simulink model "AdaptiveOb"  (R2019b)
settings: Solver=VariableStepAuto  StartTime=0.0  StopTime=10.0  RelTol=1e-3
undefined symbols (not defined in the file): DiscIntNeverNeededParam, INJ_FRQ, J, KLdd, KLgd, KLgg, KR, Ldq, LGammaDelta, RsRated, theta_tilde, TsimCurLoop, TsimMotor, Umdh_Cmd, Umgh_Cmd, weRated
settings Model: Creator=Downstream  LastModifiedBy=Downstream

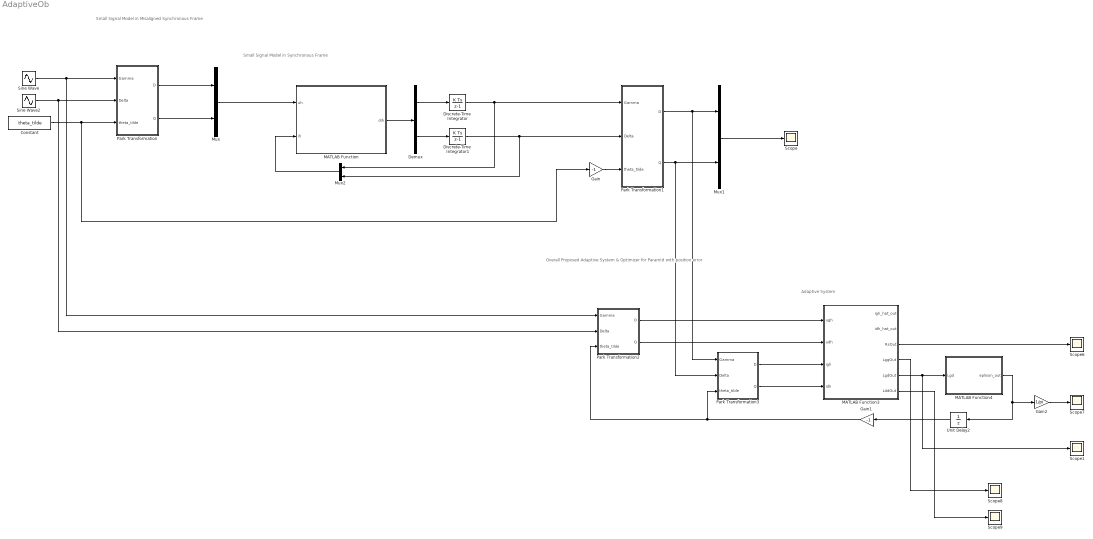
== system AdaptiveOb ==
  note: Overall Proposed Adaptive System & Optimizer for ParamId with position error
  note: Adaptive System
  note: Small Signal Model in Misaligned Synchronous Frame
  note: Small Signal Model in Synchronous Frame
  Constant : Constant  Value=theta_tilde  SampleTime=TsimMotor
  Demux : Demux  Outputs=2
  Discrete-Time Integrator : DiscreteIntegrator  Priority=1  SampleTime=-1  ICPrevOutput=DiscIntNeverNeededParam  ICPrevScaledInput=DiscIntNeverNeededParam
  Discrete-Time Integrator1 : DiscreteIntegrator  Priority=1  SampleTime=-1  ICPrevOutput=DiscIntNeverNeededParam  ICPrevScaledInput=DiscIntNeverNeededParam
  Gain : Gain  Gain=-1
  Gain1 : Gain  Gain=-1
  Gain2 : Gain  Gain=1/pi
  MATLAB Function : MATLAB Function  TreatAsAtomicUnit=on
  MATLAB Function3 : MATLAB Function  Priority=9  TreatAsAtomicUnit=on  SystemSampleTime=TsimCurLoop
  MATLAB Function4 : MATLAB Function  TreatAsAtomicUnit=on
  Mux : Mux  Inputs=2
  Mux1 : Mux  Inputs=2
  Mux2 : Mux  Inputs=2
  Park Transformation : Subsystem
  Park Transformation1 : Subsystem
  Park Transformation2 : Subsystem
  Park Transformation3 : Subsystem
  Scope{,1,6..9} (6 alike) : Scope
  Sine Wave : Sin  Priority=4  Amplitude=Umgh_Cmd  Frequency=INJ_FRQ * 2 * pi  SampleTime=TsimCurLoop
  Sine Wave2 : Sin  Priority=5  Amplitude=Umdh_Cmd  Frequency=INJ_FRQ * 2 * pi  Phase=pi/2  SampleTime=TsimCurLoop
  Unit Delay2 : UnitDelay  SampleTime=-1  HasFrameUpgradeWarning=on
  wires:
  Constant/1 -> Park Transformation/3(theta_tilde), Gain/1
  Mux/1 -> MATLAB Function/1(uh)
  MATLAB Function/1(dih) -> Demux/1
  Demux/1 -> Discrete-Time Integrator/1
  Demux/2 -> Discrete-Time Integrator1/1
  Gain/1 -> Park Transformation1/3(theta_tilde)
  Mux1/1 -> Scope/1
  Park Transformation/1(D) -> Mux/1
  Park Transformation/2(Q) -> Mux/2
  Discrete-Time Integrator1/1 -> Park Transformation1/2(Delta), Mux2/2
  Discrete-Time Integrator/1 -> Mux2/1, Park Transformation1/1(Gamma)
  Mux2/1 -> MATLAB Function/2(ih)
  Park Transformation3/1(D) -> MATLAB Function3/3(igh)
  Park Transformation3/2(Q) -> MATLAB Function3/4(idh)
  MATLAB Function3/5(LgdOut) -> Scope1/1, MATLAB Function4/1(Lgd)
  MATLAB Function4/1(eplison_out) -> Gain2/1, Unit Delay2/1
  Gain1/1 -> Park Transformation3/3(theta_tilde), Park Transformation2/3(theta_tilde)
  MATLAB Function3/3(RsOut) -> Scope6/1
  Unit Delay2/1 -> Gain1/1
  Gain2/1 -> Scope7/1
  Sine Wave/1 -> Park Transformation2/1(Gamma), Park Transformation/1(Gamma)
  Sine Wave2/1 -> Park Transformation2/2(Delta), Park Transformation/2(Delta)
  MATLAB Function3/4(LggOut) -> Scope8/1
  MATLAB Function3/6(LddOut) -> Scope9/1
  Park Transformation1/1(D) -> Park Transformation3/1(Gamma), Mux1/1
  Park Transformation1/2(Q) -> Mux1/2, Park Transformation3/2(Delta)
  Park Transformation2/1(D) -> MATLAB Function3/1(ugh)
  Park Transformation2/2(Q) -> MATLAB Function3/2(udh)

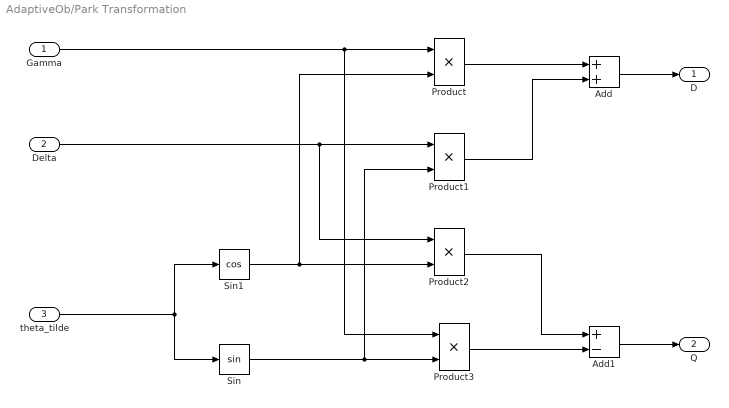
== system AdaptiveOb/Park Transformation ==
  Gamma : Inport
  Delta : Inport  Port=2
  theta_tilde : Inport  Port=3
  Add : Sum
  Add1 : Sum  Inputs=+-
  Product{,1..3} (4 alike) : Product
  Sin : Trigonometry  OutputSignalType=real
  Sin1 : Trigonometry  Operator=cos  OutputSignalType=real
  D : Outport
  Q : Outport  Port=2
  wires:
  Product/1 -> Add/1
  Sin/1 -> Product3/2, Product1/2
  Product1/1 -> Add/2
  Add1/1 -> Q/1
  Sin1/1 -> Product2/2, Product/2
  Product2/1 -> Add1/1
  Gamma/1 -> Product3/1, Product/1
  Delta/1 -> Product2/1, Product1/1
  Product3/1 -> Add1/2
  Add/1 -> D/1
  theta_tilde/1 -> Sin/1, Sin1/1

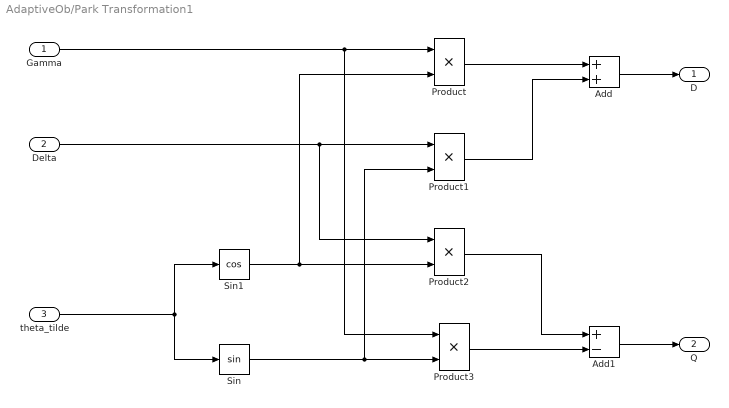
== system AdaptiveOb/Park Transformation1 ==
  Gamma : Inport
  Delta : Inport  Port=2
  theta_tilde : Inport  Port=3
  Add : Sum
  Add1 : Sum  Inputs=+-
  Product{,1..3} (4 alike) : Product
  Sin : Trigonometry  OutputSignalType=real
  Sin1 : Trigonometry  Operator=cos  OutputSignalType=real
  D : Outport
  Q : Outport  Port=2
  wires:
  Product/1 -> Add/1
  Sin/1 -> Product3/2, Product1/2
  Product1/1 -> Add/2
  Add1/1 -> Q/1
  Sin1/1 -> Product2/2, Product/2
  Product2/1 -> Add1/1
  Gamma/1 -> Product3/1, Product/1
  Delta/1 -> Product2/1, Product1/1
  Product3/1 -> Add1/2
  Add/1 -> D/1
  theta_tilde/1 -> Sin/1, Sin1/1

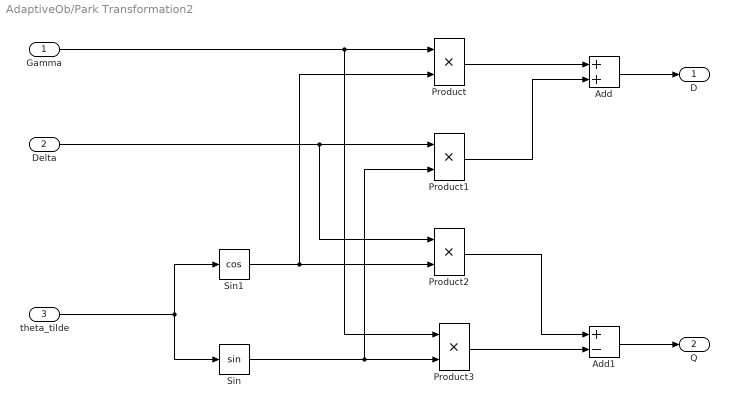
== system AdaptiveOb/Park Transformation2 ==
  Gamma : Inport
  Delta : Inport  Port=2
  theta_tilde : Inport  Port=3
  Add : Sum
  Add1 : Sum  Inputs=+-
  Product{,1..3} (4 alike) : Product
  Sin : Trigonometry  OutputSignalType=real
  Sin1 : Trigonometry  Operator=cos  OutputSignalType=real
  D : Outport
  Q : Outport  Port=2
  wires:
  Product/1 -> Add/1
  Sin/1 -> Product3/2, Product1/2
  Product1/1 -> Add/2
  Add1/1 -> Q/1
  Sin1/1 -> Product2/2, Product/2
  Product2/1 -> Add1/1
  Gamma/1 -> Product3/1, Product/1
  Delta/1 -> Product2/1, Product1/1
  Product3/1 -> Add1/2
  Add/1 -> D/1
  theta_tilde/1 -> Sin/1, Sin1/1

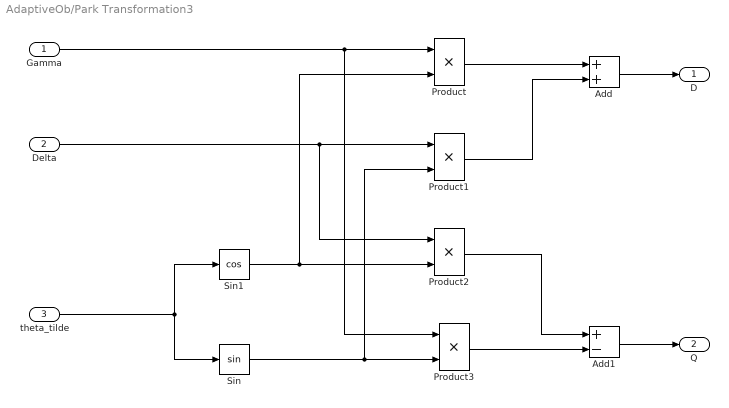
== system AdaptiveOb/Park Transformation3 ==
  Gamma : Inport
  Delta : Inport  Port=2
  theta_tilde : Inport  Port=3
  Add : Sum
  Add1 : Sum  Inputs=+-
  Product{,1..3} (4 alike) : Product
  Sin : Trigonometry  OutputSignalType=real
  Sin1 : Trigonometry  Operator=cos  OutputSignalType=real
  D : Outport
  Q : Outport  Port=2
  wires:
  theta_tilde/1 -> Sin1/1, Sin/1
  Add/1 -> D/1
  Product3/1 -> Add1/2
  Delta/1 -> Product1/1, Product2/1
  Gamma/1 -> Product/1, Product3/1
  Product2/1 -> Add1/1
  Sin1/1 -> Product/2, Product2/2
  Add1/1 -> Q/1
  Product1/1 -> Add/2
  Sin/1 -> Product1/2, Product3/2
  Product/1 -> Add/1

== matlab function AdaptiveOb/MATLAB Function ==
  data: uh input; dih output; ih input; RsRated parameter; Ldq parameter; J parameter; weRated parameter
function dih  = SmallSignalModel(uh,ih,RsRated, Ldq, J, weRated)
A = -(RsRated + weRated * J * Ldq);
dih = A * ih + uh;
dih = Ldq^-1 * dih;

== matlab function AdaptiveOb/MATLAB Function3 ==
  data: ugh input; udh input; igh_hat_out output; igh input; idh input; idh_hat_out output; weRated parameter; J parameter; RsRated parameter; LGammaDelta parameter; TsimCurLoop parameter; RsOut output; LggOut output; LgdOut output; LddOut output; KLgg parameter; KLgd parameter; KR parameter; KLdd parameter
function [igh_hat_out,idh_hat_out,RsOut,LggOut,LgdOut,LddOut] = AdaptiveSystem(ugh,udh,igh,idh,weRated, J, RsRated, LGammaDelta, TsimCurLoop,KLgg, KLgd, KR, KLdd)
persistent igh_hat idh_hat Rs_hat Lgg_hat Ldd_hat Lgd_hat
if isempty (igh_hat)
    igh_hat = 0;
    idh_hat = 0;
    Rs_hat = RsRated/2*2;
    Lgg_hat = LGammaDelta(1,1)/2*2;
    Ldd_hat = LGammaDelta(2,2)/2*2;
    Lgd_hat = LGammaDelta(1,2)/2*2;
end
    i_hat = [igh_hat;idh_hat;];
    i     = [igh;idh;];
    i_tilde=i_hat - i;
    igh_tilde = i_tilde(1,1);
    idh_tilde = i_tilde(2,1);
    u = [ugh;udh;];
    L_hat = [Lgg_hat Lgd_hat;Lgd_hat Ldd_hat;];
    
    i_hat_dot = (L_hat^-1) * (-(Rs_hat + weRated * J * L_hat) * i_hat + u);
    %%%%%%%%%% Calculating i_hat_new
    A = -(L_hat^-1) * (Rs_hat + weRated * J * L_hat);
    B = (L_hat^-1);
    Phi = eye(2) + TsimCurLoop * A + 0.5 * TsimCurLoop * TsimCurLoop * A * A;
    G = B * TsimCurLoop * (eye(2) + 0.5 * TsimCurLoop * A);
    i_hat_new = Phi * i_hat + G * (u - weRated * i_tilde * 0e-3);
    
    
    igh_hat_dot = i_hat_dot(1,1);
    idh_hat_dot = i_hat_dot(2,1);
%     for i = 1:2
%         if(i_hat_new(i,1)> 10)
%             i_hat_new(i,1) = 10;
%         elseif(i_hat_new(i,1) < -10)
%             i_hat_new(i,1) = -10;
%         end    
%     end
    
    Rs_hat = Rs_hat + TsimCurLoop * KR * (i_tilde' * i_hat);
    Ldd_hat = Ldd_hat + TsimCurLoop * KLdd * (-weRated * idh_hat * igh_tilde + idh_tilde * idh_hat_dot);
    Lgd_hat = Lgd_hat + TsimCurLoop * KLgd * (-weRated * igh_hat * igh_tilde + weRated * idh_hat * idh_tilde + igh_tilde * idh_hat_dot + idh_tilde * igh_hat_dot);
    Lgg_hat = Lgg_hat + TsimCurLoop * KLgg * ( weRated * igh_hat * idh_tilde + igh_tilde * igh_hat_dot);
    RsOut = Rs_hat;
    LggOut = Lgg_hat;
    LgdOut = Lgd_hat;
    LddOut = Ldd_hat;
    
    igh_hat_out = i_hat_new(1,1);
    idh_hat_out = i_hat_new(2,1);
    igh_hat = i_hat_new(1,1);
    idh_hat = i_hat_new(2,1);

== matlab function AdaptiveOb/MATLAB Function4 ==
  data: Lgd input; eplison_out output
function eplison_out = Optimizer(Lgd)
persistent eplison
if isempty(eplison)
    eplison = 0;
end
if (Lgd >0)
    eplison = eplison + 1e-5;
else
    eplison = eplison - 1e-5;
end
eplison_out = eplison;
